simulink subsystem "controller"  (R2019b)
settings: Solver=VariableStepAuto  StartTime=0.0  StopTime=10.0  RelTol=1e-3
undefined symbols (not defined in the file): K, Ts
settings Model: Creator=enrique.babio  LastModifiedBy=enrique.babio

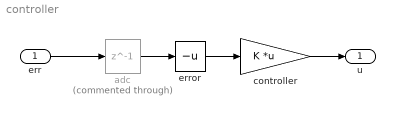
== system controller ==
  err : Inport
  adc : Delay  Commented=through  DelayLength=1  SampleTime=Ts  StateName=adcDelay
  controller : Gain  Gain=K  Multiplication=Matrix(K*u)
  error : UnaryMinus
  u : Outport
  wires:
  err/1 -> adc/1
  controller/1 -> u/1
  adc/1 -> error/1
  error/1 -> controller/1
